simulink subsystem "UserInputsOpenLoopHost"  (R2024b)
settings: Solver=VariableStepAuto  StartTime=0.0  StopTime=10.0  RelTol=1e-3
libraries: simulink x3
settings Model: Creator=The MathWorks, Inc.  LastModifiedBy=snarayan
settings RTWCC: GPUComputeCapability=3.5  LargeConstantGeneration=WriteOnlyDNNConstantsToDataFiles

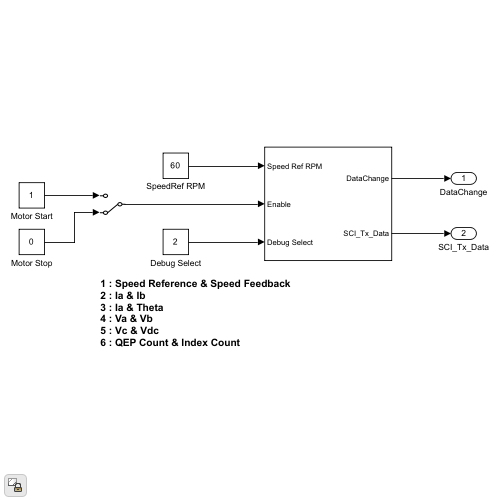
[thumbnail: Simulink's stored preview of the top-level diagram]
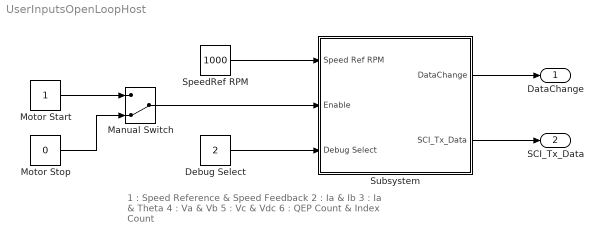
== system UserInputsOpenLoopHost ==
  note: 1 : Speed Reference & Speed Feedback
      | 2 : Ia & Ib
      | 3 : Ia & Theta
      | 4 : Va & Vb
      | 5 : Vc & Vdc
      | 6 : QEP Count & Index Count
  Debug Select : Constant  Value=2  OutDataTypeStr=uint8  SampleTime=-1
  Manual Switch : ManualSwitch  CurrentSetting=0
  Motor Start : Constant  OutDataTypeStr=uint16  SampleTime=-1
  Motor Stop : Constant  Value=0  OutDataTypeStr=uint16  SampleTime=-1
  SpeedRef RPM : Constant  Value=1000  OutDataTypeStr=int16  SampleTime=-1
  Subsystem : Subsystem
  DataChange : Outport
  SCI_Tx_Data : Outport  Port=2
  wires:
  Subsystem/1(DataChange) -> DataChange/1
  Subsystem/2(SCI_Tx_Data) -> SCI_Tx_Data/1
  SpeedRef RPM/1 -> Subsystem/1(Speed Ref RPM)
  Debug Select/1 -> Subsystem/3(Debug Select)
  Manual Switch/1 -> Subsystem/2(Enable)
  Motor Start/1 -> Manual Switch/1
  Motor Stop/1 -> Manual Switch/2

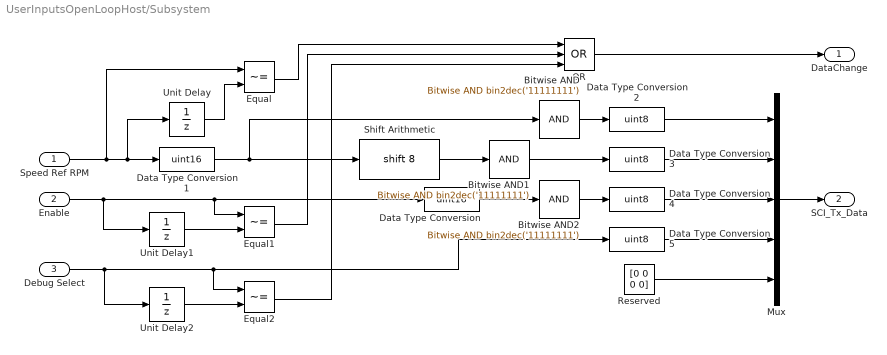
== system UserInputsOpenLoopHost/Subsystem ==
  Speed Ref RPM : Inport
  Enable : Inport  Port=2
  Debug Select : Inport  Port=3
  Bitwise AND : simulink/Logic and Bit Operations/Bitwise Operator  logicop=AND  UseBitMask=on  BitMask=bin2dec('11111111')  BitMaskRealWorld=Stored Integer
      settings: LibrarySourceBlock=|
      | simulink/Quick Insert/Logic and Bit
      | Operations/Bitwise AND
  Bitwise AND1 : simulink/Logic and Bit Operations/Bitwise Operator  logicop=AND  UseBitMask=on  BitMask=bin2dec('11111111')  BitMaskRealWorld=Stored Integer
      settings: LibrarySourceBlock=|
      | simulink/Quick Insert/Logic and Bit
      | Operations/Bitwise AND
  Bitwise AND2 : simulink/Logic and Bit Operations/Bitwise Operator  logicop=AND  UseBitMask=on  BitMask=bin2dec('11111111')  BitMaskRealWorld=Stored Integer
      settings: LibrarySourceBlock=|
      | simulink/Quick Insert/Logic and Bit
      | Operations/Bitwise AND
  Data Type Conversion : DataTypeConversion  OutDataTypeStr=uint16  ConvertRealWorld=Stored Integer (SI)  RndMeth=Simplest  SaturateOnIntegerOverflow=off
  Data Type Conversion1 : DataTypeConversion  OutDataTypeStr=uint16  ConvertRealWorld=Stored Integer (SI)  RndMeth=Simplest  SaturateOnIntegerOverflow=off
  Data Type Conversion{2..5} (4 alike) : DataTypeConversion  OutDataTypeStr=uint8  ConvertRealWorld=Stored Integer (SI)  RndMeth=Simplest  SaturateOnIntegerOverflow=off
  Equal : RelationalOperator  Operator=~=  OutDataTypeStr=boolean  RndMeth=Simplest  InputSameDT=off
  Equal1 : RelationalOperator  Operator=~=  OutDataTypeStr=boolean  RndMeth=Simplest  InputSameDT=off
  Equal2 : RelationalOperator  Operator=~=  OutDataTypeStr=boolean  RndMeth=Simplest  InputSameDT=off
  Mux : Mux  Inputs=5
  OR : Logic  Operator=OR  Inputs=3  IconShape=distinctive  AllPortsSameDT=off  OutDataTypeStr=boolean
  Reserved : Constant  Value=[0 0 0 0]  OutDataTypeStr=uint8  SampleTime=-1
  Shift Arithmetic : ArithShift  BitShiftNumber=8
  Unit Delay : UnitDelay  SampleTime=-1  HasFrameUpgradeWarning=on
  Unit Delay1 : UnitDelay  SampleTime=-1  HasFrameUpgradeWarning=on
  Unit Delay2 : UnitDelay  SampleTime=-1  HasFrameUpgradeWarning=on
  DataChange : Outport
  SCI_Tx_Data : Outport  Port=2
  wires:
  Unit Delay2/1 -> Equal2/2
  Equal2/1 -> OR/3
  Reserved/1 -> Mux/5
  Data Type Conversion3/1 -> Mux/2
  Data Type Conversion5/1 -> Mux/4
  Data Type Conversion2/1 -> Mux/1
  Debug Select/1 -> Data Type Conversion5/1, Equal2/1, Unit Delay2/1
  Data Type Conversion4/1 -> Mux/3
  Bitwise AND1/1 -> Data Type Conversion3/1
  Bitwise AND/1 -> Data Type Conversion2/1
  Bitwise AND2/1 -> Data Type Conversion4/1
  Equal1/1 -> OR/2
  Data Type Conversion1/1 -> Bitwise AND/1, Shift Arithmetic/1
  Unit Delay1/1 -> Equal1/2
  Shift Arithmetic/1 -> Bitwise AND1/1
  Data Type Conversion/1 -> Bitwise AND2/1
  Equal/1 -> OR/1
  OR/1 -> DataChange/1
  Enable/1 -> Equal1/1, Data Type Conversion/1, Unit Delay1/1
  Mux/1 -> SCI_Tx_Data/1
  Unit Delay/1 -> Equal/2
  Speed Ref RPM/1 -> Equal/1, Unit Delay/1, Data Type Conversion1/1
